simulink library "sensor_bus"  (R2018b)
settings: Solver=VariableStepAuto  StartTime=0.0  StopTime=10.0  RelTol=1e-3
undefined symbols (not defined in the file): simParams
settings Model: Creator=satcave1  LastModifiedBy=taylorreynolds

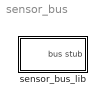
== system sensor_bus ==
  sensor_bus_lib : Subsystem

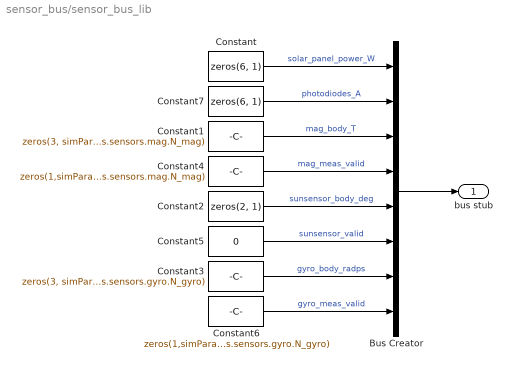
== system sensor_bus/sensor_bus_lib ==
  Bus Creator : BusCreator  Inputs=8
  Constant : Constant  Value=zeros(6, 1)
  Constant1 : Constant  Value=zeros(3, simParams.sensors.mag.N_mag)
  Constant2 : Constant  Value=zeros(2, 1)
  Constant3 : Constant  Value=zeros(3, simParams.sensors.gyro.N_gyro)
  Constant4 : Constant  Value=zeros(1,simParams.sensors.mag.N_mag)  OutDataTypeStr=boolean
  Constant5 : Constant  Value=0  OutDataTypeStr=boolean
  Constant6 : Constant  Value=zeros(1,simParams.sensors.gyro.N_gyro)  OutDataTypeStr=boolean
  Constant7 : Constant  Value=zeros(6, 1)
  bus stub : Outport
  wires:
  Constant2/1 -> Bus Creator/5  "sunsensor_body_deg"
  Bus Creator/1 -> bus stub/1
  Constant3/1 -> Bus Creator/7  "gyro_body_radps"
  Constant/1 -> Bus Creator/1  "solar_panel_power_W"
  Constant4/1 -> Bus Creator/4  "mag_meas_valid"
  Constant1/1 -> Bus Creator/3  "mag_body_T"
  Constant6/1 -> Bus Creator/8  "gyro_meas_valid"
  Constant5/1 -> Bus Creator/6  "sunsensor_valid"
  Constant7/1 -> Bus Creator/2  "photodiodes_A"
